simulink model "sensors"  (R2022a)
settings: Solver=VariableStepAuto  StartTime=0.0  StopTime=10.0  RelTol=1e-3
undefined symbols (not defined in the file): gray
libraries: sim3dcameralib x1, sim3dphyssensorlib x1, sim3dprobsensorlib x1, sim3dlib x1
settings Model: Creator=mccat  LastModifiedBy=mccat

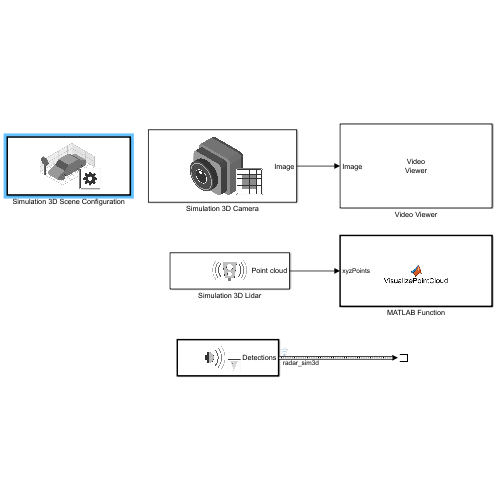
[thumbnail: Simulink's stored preview of the top-level diagram]
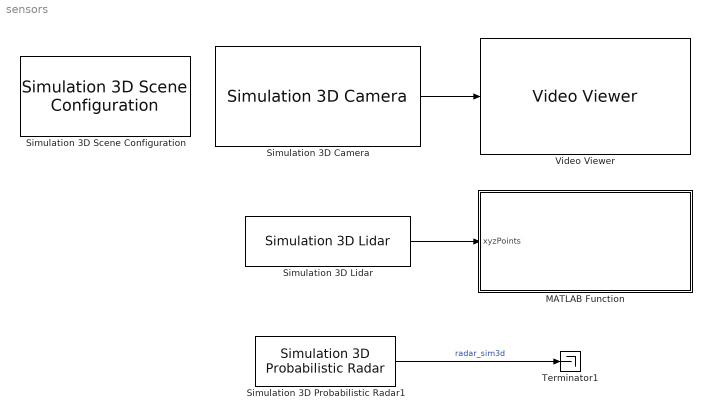
== system sensors ==
  MATLAB Function : MATLAB Function  TreatAsAtomicUnit=on
  Simulation 3D Camera : sim3dcameralib/Simulation 3D Camera  Priority=1  sensorTag=Sim3dSensor1  sensorId=1  sensorName=Sim3dSensor1  vehTagList={'Scene Origin'}  vehTag=Scene Origin  mountLoc=Origin  offsetFlag=on  tmountOffset=[0.57, 0, 1.2]  extTmount=off  rmountOffset=[0, 0, 0]  extRmount=off  FocalLength=[1109, 1109]  OpticalCenter=[640, 360]  ImageSize=[720, 1280]  RadialDistortion=[0, 0]  TangentialDistortion=[0, 0]  SensorSkew=0  DepthOutportEnabled=off  SemanticOutportEnabled=off  TransformOutportEnabled=off  SampleTime=-1  mountPoint=[0.57 0 1.2]  mountOrientation=[0 0 0]  aMode=3  ID=1
      settings: SourceProductBaseCode=VE,AE,DR,UV,VE
  Simulation 3D Lidar : sim3dphyssensorlib/Simulation 3D Lidar  Priority=1  sensorTag=Sim3dSensor2  sensorId=2  sensorName=Sim3dSensor2  vehTagList={'Scene Origin'}  vehTag=Scene Origin  mountLoc=Origin  offsetFlag=off  tmountOffset=[0, 0, 0]  rmountOffset=[0, 0, 0]  DetectionRange=120  RangeResolution=0.002  VerticalFOV=40  VerticalResolution=1.25  HorizontalFOV=360  HorizontalResolution=0.16  DistanceOutportEnabled=off  ReflectivityOutportEnabled=off  TransformOutportEnabled=off  SampleTime=-1  mountPoint=[0 0 0]  mountOrientation=[0 0 0]  aMode=3  ID=2
      settings: SourceProductBaseCode=VE,AE,DR,UV,VE
  Simulation 3D Probabilistic Radar1 : sim3dprobsensorlib/Simulation 3D Probabilistic Radar  Priority=1  sensorTag=Sim3dSensor3  sensorId=3  sensorName=Sim3dSensor3  vehTagList={'Scene Origin'}  vehTag=Scene Origin  mountLoc=Origin  offsetFlag=off  tmountOffset=[0, 0, 0]  rmountOffset=[0, 0, 0]  AzimuthResolution=4  ElevationResolution=10  RangeResolution=2.5  RangeRateResolution=0.5  AzimuthBiasFraction=0.1  ElevationBiasFraction=0.1  RangeBiasFraction=0.05  RangeRateBiasFraction=0.05  FieldOfView=[ 20, 5 ]  DetectionRange=[ 1, 150 ]  RangeRateLimits=[ -100, 100 ]  DetectionProbability=0.9  FalseAlarmRate=1e-6  ReferenceRange=100  ReferenceRCS=0  HasElevation=on  HasRangeRate=on  HasNoise=on  HasFalseAlarms=on  InitialSeedSource=Repeatable  InitialSeed=0  MaxNumDetections=50  DetectionCoordinates=Ego Cartesian  SpecifyOutputBusName=off  BusName=BusSimulation3DRadarTruthSensor  SampleTime=-1  mountPoint=[0 0 0]  mountOrientation=[0 0 0]  aMode=3  ID=3
      settings: SourceProductBaseCode=VE,AE,DR,UV,VE
  Simulation 3D Scene Configuration : sim3dlib/Simulation 3D Scene Configuration  Priority=0  ProjectFormat=Unreal Executable  SceneDesc=Curved road  ProjectName=C:\ProgramData\MATLAB\SupportPackages\R2022a\toolbox\shared\sim3dprojects\driving\RoadRunnerScenes\WindowsPackage\RRScene.exe  ScenePath=/Game/Maps/RRHighway  UEProjPath=F:\Kunal_Laptop_Mathworks\Unreal\Demo\HighwayLaneFollowingWithRoadRunner\RRCosim20a\RRCosim20a.uproject  vehTagList={'Scene Origin'}  vehTag=Scene Origin  OpVisEn=off  Ts=0.1  EnableWindow=on  EnableRemoteAccess=off  EnableWeather=off  SunAltitude=40.0  SunAzimuth=90  clouds=10  wind=1  fog=0  rain=0  sensorTag=MainCamera1  sensorId=1  sensorName=MainCamera1  mountLoc=Origin  offsetFlag=off  tmountOffset=[0, 0, 0]  rmountOffset=[0, 0, 0]  HorizontalResolution=1280  VerticalResolution=720  HorizontalFOV=60  mountPoint=[0 0 0]  mountOrientation=[0 0 0]  aMode=3  ID=1
      settings: SourceProductBaseCode=VE,AE,DR,UV,VE
  Terminator1 : Terminator
  Video Viewer : VideoViewer  colormapValue=gray(256)  FigPos=[-4.33333333333333 515.333333333333 430 322.666666666667]  OpenAtMdlStart=off
  wires:
  Simulation 3D Camera/1 -> Video Viewer/1
  Simulation 3D Probabilistic Radar1/1 -> Terminator1/1  "radar_sim3d"
  Simulation 3D Lidar/1 -> MATLAB Function/1(xyzPoints)

== matlab function sensors/MATLAB Function ==
  data: xyzPoints input
function VisualizePointCloud(xyzPoints)
%VisualizePointCloud Display point cloud

coder.extrinsic('isOpen', 'pcplayer')

persistent player;

if isempty(player)
    % Configure axes limits
    xlimits = [-90 90];
    ylimits = [-90 90];
    zlimits = [ -5 40];
    
    % Create a streaming Lidar viewer
    player = pcplayer(xlimits, ylimits, zlimits);
end

if ~isempty(player) && isOpen(player)
    view(player, xyzPoints);
end
